simulink model "off_grid_RRC"  (R2015b)
settings: Solver=ode45  StartTime=0.0  StopTime=5  RelTol=1e-3
libraries: powerlib x55, powerlib_meascontrol x6, powerlib_extras x6
settings Model: Creator=Pouyan  LastModifiedBy=fujitsu
settings DataIOCC: SaveFormat=Array  SignalLoggingSaveFormat=ModelDataLogs
settings OptimizationCC: ExpressionDepthLimit=2147483647
settings DebuggingCC: UnderspecifiedInitializationDetection=Classic  MergeDetectMultiDrivingBlocksExec=none  SolverPrmCheckMsg=warning  FcnCallInpInsideContextMsg=UseLocalSettings  StateNameClashWarn=warning
settings HardwareCC: ProdBitPerPointer=32  ProdLargestAtomicFloat=None  ProdIntDivRoundTo=Undefined  ProdEndianess=Unspecified  ProdWordSize=32  ProdHWDeviceType=32-bit Generic
settings GRTTargetCC: GeneratePreprocessorConditionals=Disable all  CombineOutputUpdateFcns=off  GRTInterface=on
settings ConfigComp: CovModelRefEnable=Off

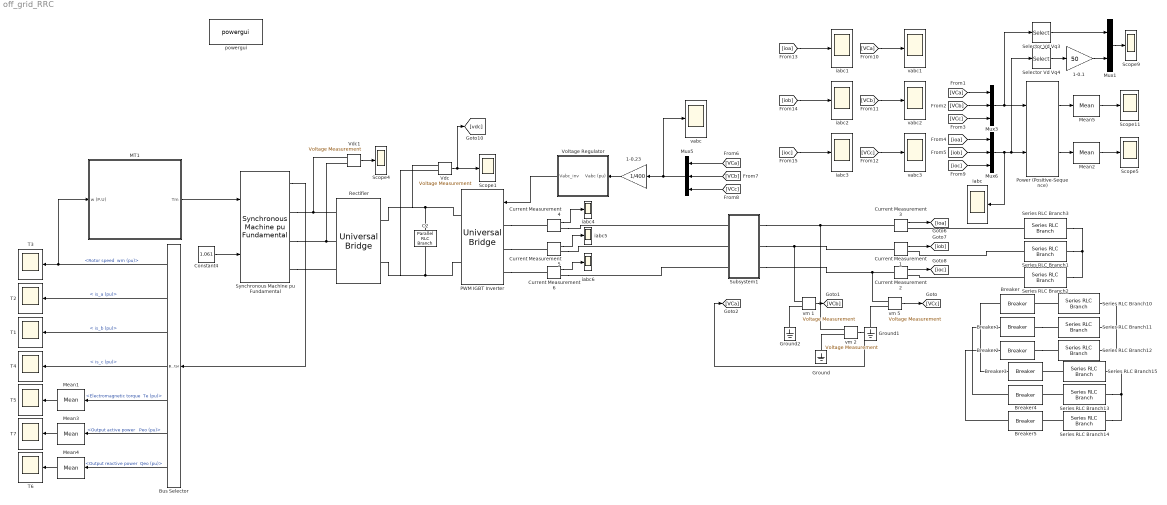
== system off_grid_RRC ==
  1-0.1 : Gain  Gain=50
  1-0.23 : Gain  Gain=1/400
  Breaker : powerlib/Elements/Breaker  InitialState=0  SwitchingTimes=[4 8]  External=off  BreakerResistance=0.01  SnubberResistance=1e6  SnubberCapacitance=inf  Measurements=None  MoreParameters=on  NoBreakLoop=off
  Breaker1 : powerlib/Elements/Breaker  InitialState=0  SwitchingTimes=[4 8]  External=off  BreakerResistance=0.01  SnubberResistance=1e6  SnubberCapacitance=inf  Measurements=None  MoreParameters=on  NoBreakLoop=off
  Breaker2 : powerlib/Elements/Breaker  InitialState=0  SwitchingTimes=[4 8]  External=off  BreakerResistance=0.01  SnubberResistance=1e6  SnubberCapacitance=inf  Measurements=None  MoreParameters=on  NoBreakLoop=off
  Breaker3 : powerlib/Elements/Breaker  InitialState=0  SwitchingTimes=[6 8.5]  External=off  BreakerResistance=0.01  SnubberResistance=1e6  SnubberCapacitance=inf  Measurements=None  MoreParameters=on  NoBreakLoop=off
  Breaker4 : powerlib/Elements/Breaker  InitialState=0  SwitchingTimes=[6 8.5]  External=off  BreakerResistance=0.01  SnubberResistance=1e6  SnubberCapacitance=inf  Measurements=None  MoreParameters=on  NoBreakLoop=off
  Breaker5 : powerlib/Elements/Breaker  InitialState=0  SwitchingTimes=[6 8.5]  External=off  BreakerResistance=0.01  SnubberResistance=1e6  SnubberCapacitance=inf  Measurements=None  MoreParameters=on  NoBreakLoop=off
  Bus Selector : BusSelector  OutputSignals="Mechanical.Rotor speed  wm (pu),Stator current. is_a (pu),Stator current. is_b (pu),Stator current. is_c (pu),Mechanical.Electromagnetic torque  Te (pu),Output active power   Peo (pu),Output reactive power  Qeo (pu)"
  C2 : powerlib/Elements/Parallel RLC Branch  LConnTagsString=a  RConnTagsString=__new0  BranchType=C  Resistance=inf  Inductance=inf  SetiL0=off  InitialCurrent=0  Capacitance=5000e-06  Setx0=off  InitialVoltage=0  Measurements=None
  Constant4 : Constant  Value=1.061
  Current Measurement{1..6} (6 alike) : powerlib/Measurements/Current Measurement  PhasorSimulation=off  OutputType=Complex  PSBequivalent=0
  Ground : powerlib/Elements/Ground  LConnTagsString=a
  Ground1 : powerlib/Elements/Ground  LConnTagsString=a
  Ground2 : powerlib/Elements/Ground  LConnTagsString=a
  MT1 : Subsystem
  Mean{1..5} (5 alike) : powerlib_meascontrol/Measurements/Mean  Freq=50  Vinit=0  Ts=5e-6
  Mux1 : Mux  Inputs=2
  Mux3 : Mux  Inputs=3
  Mux5 : Mux  Inputs=3
  Mux6 : Mux  Inputs=3
  PWM IGBT Inverter : powerlib/Power Electronics/Universal Bridge  Arms=3  SnubberResistance=5000  SnubberCapacitance=inf  Device=IGBT / Diodes  Ron=1e-3  Lon=0  ForwardVoltages="[  0.0  0.0  ]"  ForwardVoltage=.8  GTOparameters=[ 1e-6 ,1e-6 ]  IGBTparameters=[ 1e-6 , 2e-6 ]  Measurements=Device currents  Measurements_2=None  converterType=Rectifier
  Power (Positive-Sequence) : powerlib_meascontrol/Measurements/Power (Positive-Sequence)  Freq=50  Vinit=[0, 0]  Iinit=[0, 0]  Ts=5e-6
  Rectifier : powerlib/Power Electronics/Universal Bridge  Arms=3  SnubberResistance=50  SnubberCapacitance=0.1e-6  Device=Diodes  Ron=1e-3  Lon=0  ForwardVoltages="[  0.8  0.8  ]"  ForwardVoltage=.7  GTOparameters=[ 10e-6 , 20e-6 ]  IGBTparameters=[ 1e-6 , 2e-6 ]  Measurements=Device currents  Measurements_2=None  converterType=Rectifier
  Scope{1,4..5,9,11} (5 alike) : Scope
  Selector Vd Vq3 : Selector  InputPortWidth=3  IndexOptions=Index vector (dialog)  Indices=[1]  OutputSizes=1
  Selector Vd Vq4 : Selector  InputPortWidth=3  IndexOptions=Index vector (dialog)  Indices=[1]  OutputSizes=1
  Series RLC Branch1 : powerlib/Elements/Series RLC Branch  LConnTagsString=__new0  RConnTagsString=__new0  BranchType=RL  Resistance=50  Inductance=100e-3  SetiL0=off  InitialCurrent=0  Capacitance=1e-6  Setx0=off  InitialVoltage=0  Measurements=None
  Series RLC Branch10 : powerlib/Elements/Series RLC Branch  LConnTagsString=__new0  RConnTagsString=__new0  BranchType=RL  Resistance=50*2  Inductance=100e-3*2  SetiL0=off  InitialCurrent=0  Capacitance=1e-6  Setx0=off  InitialVoltage=0  Measurements=None
  Series RLC Branch11 : powerlib/Elements/Series RLC Branch  LConnTagsString=__new0  RConnTagsString=__new0  BranchType=RL  Resistance=50*2  Inductance=100e-3*2  SetiL0=off  InitialCurrent=0  Capacitance=1e-6  Setx0=off  InitialVoltage=0  Measurements=None
  Series RLC Branch12 : powerlib/Elements/Series RLC Branch  LConnTagsString=__new0  RConnTagsString=__new0  BranchType=RL  Resistance=50*2  Inductance=100e-3*2  SetiL0=off  InitialCurrent=0  Capacitance=1e-6  Setx0=off  InitialVoltage=0  Measurements=None
  Series RLC Branch13 : powerlib/Elements/Series RLC Branch  LConnTagsString=__new0  RConnTagsString=__new0  BranchType=RL  Resistance=50*3  Inductance=(100e-3)*3  SetiL0=off  InitialCurrent=0  Capacitance=1e-6  Setx0=off  InitialVoltage=0  Measurements=None
  Series RLC Branch14 : powerlib/Elements/Series RLC Branch  LConnTagsString=__new0  RConnTagsString=__new0  BranchType=RL  Resistance=50*3  Inductance=(100e-3)*3  SetiL0=off  InitialCurrent=0  Capacitance=1e-6  Setx0=off  InitialVoltage=0  Measurements=None
  Series RLC Branch15 : powerlib/Elements/Series RLC Branch  LConnTagsString=__new0  RConnTagsString=__new0  BranchType=RL  Resistance=50*3  Inductance=(100e-3)*3  SetiL0=off  InitialCurrent=0  Capacitance=1e-6  Setx0=off  InitialVoltage=0  Measurements=None
  Series RLC Branch2 : powerlib/Elements/Series RLC Branch  LConnTagsString=__new0  RConnTagsString=__new0  BranchType=RL  Resistance=50  Inductance=100e-3  SetiL0=off  InitialCurrent=0  Capacitance=1e-6  Setx0=off  InitialVoltage=0  Measurements=None
  Series RLC Branch3 : powerlib/Elements/Series RLC Branch  LConnTagsString=__new0  RConnTagsString=__new0  BranchType=RL  Resistance=50  Inductance=100e-3  SetiL0=off  InitialCurrent=0  Capacitance=1e-6  Setx0=off  InitialVoltage=0  Measurements=None
  Subsystem1 : Subsystem
  Synchronous Machine pu Fundamental : powerlib/Machines/Synchronous Machine pu Fundamental  PresetModel=No  MechanicalLoad=Mechanical power Pm  ShowDetailedParameters=on  RotorType=Salient-pole  Units=per unit fundamental parameters  MeasurementBus=off  NominalParameters="[ 30e3  550 1600]"  Stator="[ 0.2503  0.114  0.6875  0.6875 ]"  Field="[ 1  10e15/(100*pi)]"  Dampers2=[0.0652, 0.5134, 0.0287, 0.2553, 7.765e-3, 0.9167 ]  Dampers1="[ 1.17E-02  0.182  1.97E-02  0.384 ]"  Mechanical=[ 6 0 2]  PolePairs=20  InitialConditions="[ 0  0  0  0  0  0  0  0  1 ]"  SetSaturation=off  Saturation=[0.6404,0.7127,0.8441,0.9214,0.9956,1.082,1.19,1.316,1.457;0.7,0.7698,0.8872,0.9466,0.9969,1.046,1.1,1.151,1.201]  LoadFlowParameters=[1,0,0,0,0]  TsPowergui=0  TsBlock=-1  IterativeModel=Trapezoidal non iterative  BusType=swing  Pref=0  Qref=0  Qmin=-inf  Qmax=inf  PLF=0  QLF=0
  T{1..7} (7 alike) : Scope
  Vdc : powerlib/Measurements/Voltage Measurement  Tag=PoWeRsYsTeMmEaSuReMeNt  PhasorSimulation=off  OutputType=Magnitude  PSBequivalent=0
  Vdc1 : powerlib/Measurements/Voltage Measurement  Tag=PoWeRsYsTeMmEaSuReMeNt  PhasorSimulation=off  OutputType=Magnitude  PSBequivalent=0
  Voltage Regulator : Subsystem  mask{kp=0.0001, ki=5}
  iabc{,1..6} (7 alike) : Scope
  powergui : powerlib/powergui  SimulationMode=Discrete  SolverType=Tustin  SampleTime=5e-6  frequency=60  SPID=off  DisableSnubberDevices=off  DisableRonSwitches=off  DisableVfSwitches=off  SwTol=0  DisplayEquations=off  Interpol=off  ExternalGateDelay=off  methode=off  Ts=0  FunctionMessages=off  echomessages=off  HookPort=off  EnableUseOfTLC=off  x0status=blocks  frequencyindice=0  Pbase=100e6  ErrMax=0.0001  Iterations=50  UnitsV=kV  UnitsW=MW  buscounter=0  RestoreLinks=warning  ResistiveCurrentMeasurement=off  Frange=[0:2:500]  Ylog=off  Xlog=on  ShowGrid=off  save=off  variable=ZData  structure=Vs  ZoomFFT=on  StartTime=1/60  cycles=1  DisplayStyle=1  fundamental=60  FreqAxis=on  MaxFrequency=10000  frequencyindicesteady=1  RmsSteady=1  display=off
  vabc{,1..3} (4 alike) : Scope
  vm 1 : powerlib/Measurements/Voltage Measurement  PhasorSimulation=off  OutputType=Complex  PSBequivalent=0
  vm 2 : powerlib/Measurements/Voltage Measurement  PhasorSimulation=off  OutputType=Complex  PSBequivalent=0
  vm 5 : powerlib/Measurements/Voltage Measurement  PhasorSimulation=off  OutputType=Complex  PSBequivalent=0
  wires:
  Power (Positive-Sequence)/1 -> Mean5/1
  Mean5/1 -> Scope11/1
  Mean2/1 -> Scope5/1
  MT1/1(Tm) -> Synchronous Machine pu Fundamental/1
  Synchronous Machine pu Fundamental/1 -> Bus Selector/1
  Constant4/1 -> Synchronous Machine pu Fundamental/2
  Vdc1/1 -> Scope4/1
  Vdc/1 -> [vdc], Scope1/1
  Voltage Regulator/1(Vabc_inv) -> PWM IGBT Inverter/1
  Mux1/1 -> Scope9/1
  Selector Vd Vq3/1 -> Mux1/1
  Mean4/1 -> T6/1
  Bus Selector/1 -> MT1/1(w (P.U)), T3/1  "<Rotor speed  wm (pu)>"
  Bus Selector/2 -> T2/1  "< is_a (pu)>"
  Bus Selector/3 -> T1/1  "< is_b (pu)>"
  Bus Selector/4 -> T4/1  "< is_c (pu)>"
  Bus Selector/5 -> Mean1/1  "<Electromagnetic torque  Te (pu)>"
  Mean1/1 -> T5/1
  Bus Selector/7 -> Mean4/1  "<Output reactive power  Qeo (pu)>"
  Bus Selector/6 -> Mean3/1  "<Output active power   Peo (pu)>"
  Mean3/1 -> T7/1
  Power (Positive-Sequence)/2 -> Mean2/1
  vm 5/1 -> [VCc]
  vm 1/1 -> [VCb]
  vm 2/1 -> [VCa]
  Current Measurement2/1 -> [ioc]
  1-0.23/1 -> Voltage Regulator/1(Vabc (pu))
  [VCa] -> Mux5/1
  [VCb] -> Mux5/2
  [VCc] -> Mux5/3
  Mux5/1 -> vabc/1, 1-0.23/1
  [VCc] -> Mux3/3
  [VCa] -> Mux3/1
  [VCb] -> Mux3/2
  Mux3/1 -> Selector Vd Vq3/1, Power (Positive-Sequence)/1
  [ioa] -> Mux6/1
  [iob] -> Mux6/2
  [ioc] -> Mux6/3
  Mux6/1 -> iabc/1, Selector Vd Vq4/1, Power (Positive-Sequence)/2
  Current Measurement1/1 -> [iob]
  Current Measurement3/1 -> [ioa]
  [VCa] -> vabc1/1
  [VCb] -> vabc2/1
  [VCc] -> vabc3/1
  [ioa] -> iabc1/1
  [iob] -> iabc2/1
  [ioc] -> iabc3/1
  Current Measurement4/1 -> iabc4/1
  Current Measurement5/1 -> iabc5/1
  Current Measurement6/1 -> iabc6/1
  Selector Vd Vq4/1 -> 1-0.1/1
  1-0.1/1 -> Mux1/2
  connections:
  Synchronous Machine pu Fundamental/RConn1 -- Vdc1/LConn1 -- Rectifier/LConn1
  Synchronous Machine pu Fundamental/RConn2 -- Rectifier/LConn2 -- Vdc1/LConn2
  Synchronous Machine pu Fundamental/RConn3 -- Rectifier/LConn3
  Series RLC Branch3/RConn1 -- Series RLC Branch2/RConn1 -- Series RLC Branch1/RConn1
  Series RLC Branch10/RConn1 -- Series RLC Branch12/RConn1 -- Series RLC Branch11/RConn1
  Series RLC Branch3/LConn1 -- Current Measurement3/RConn1
  Series RLC Branch1/LConn1 -- Current Measurement1/RConn1
  Series RLC Branch2/LConn1 -- Current Measurement2/RConn1
  Series RLC Branch10/LConn1 -- Breaker/RConn1
  Breaker1/RConn1 -- Series RLC Branch11/LConn1
  Breaker2/RConn1 -- Series RLC Branch12/LConn1
  Current Measurement4/RConn1 -- Subsystem1/LConn1
  PWM IGBT Inverter/LConn1 -- Current Measurement4/LConn1
  Current Measurement5/RConn1 -- Subsystem1/LConn2
  PWM IGBT Inverter/LConn2 -- Current Measurement5/LConn1
  Current Measurement6/RConn1 -- Subsystem1/LConn3
  PWM IGBT Inverter/LConn3 -- Current Measurement6/LConn1
  Series RLC Branch15/RConn1 -- Series RLC Branch14/RConn1 -- Series RLC Branch13/RConn1
  Series RLC Branch15/LConn1 -- Breaker3/RConn1
  Series RLC Branch13/LConn1 -- Breaker4/RConn1
  Series RLC Branch14/LConn1 -- Breaker5/RConn1
  Rectifier/RConn2 -- Vdc/LConn2 -- PWM IGBT Inverter/RConn2 -- C2/RConn1
  PWM IGBT Inverter/RConn1 -- Rectifier/RConn1 -- Vdc/LConn1 -- C2/LConn1
  Breaker5/LConn1 -- Breaker2/LConn1
  Breaker4/LConn1 -- Breaker1/LConn1
  Breaker/LConn1 -- Breaker3/LConn1
  Subsystem1/RConn1 -- Current Measurement3/LConn1 -- vm 2/LConn1
  Subsystem1/RConn2 -- vm 1/LConn1 -- Current Measurement1/LConn1
  Subsystem1/RConn3 -- vm 5/LConn1 -- Current Measurement2/LConn1
  vm 2/LConn2 -- Ground/LConn1
  vm 5/LConn2 -- Ground1/LConn1
  vm 1/LConn2 -- Ground2/LConn1

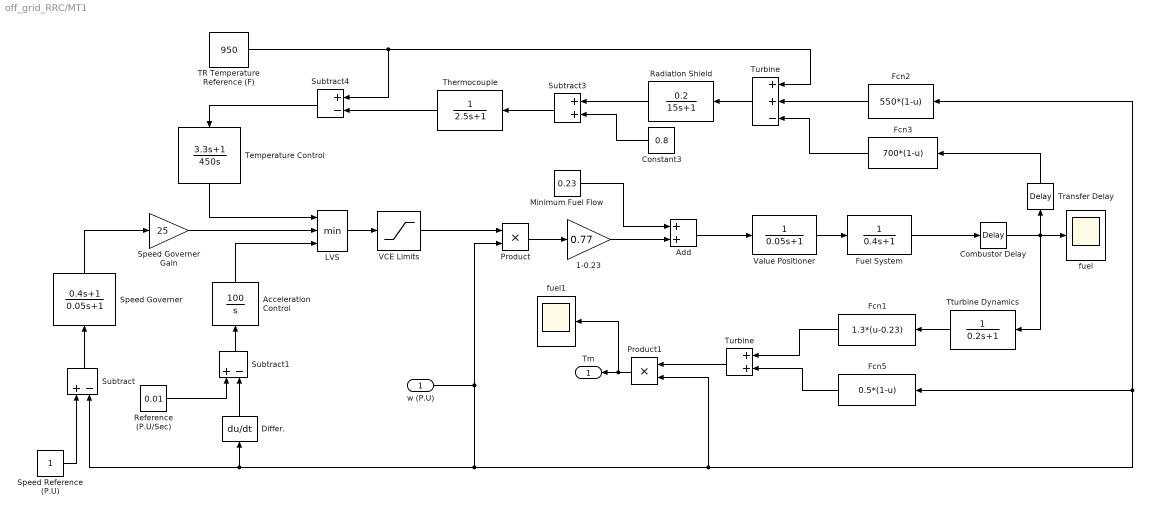
== system off_grid_RRC/MT1 ==
  w (P.U) : Inport
  1-0.23 : Gain  Gain=0.77
  Acceleration Control : TransferFcn  Numerator=[0 100]  Denominator=[1 0]
  Add : Sum
  Combustor Delay : TransportDelay  DelayTime=0.01
  Constant3 : Constant  Value=0.8
  Differ. : Derivative
  Fcn1 : Fcn  Expr=1.3*(u-0.23)
  Fcn2 : Fcn  Expr=550*(1-u)
  Fcn3 : Fcn  Expr=700*(1-u)
  Fcn5 : Fcn  Expr=0.5*(1-u)
  Fuel System : TransferFcn  Denominator=[0.4 1]
  LVS : MinMax  Inputs=3
  Minimum Fuel Flow : Constant  Value=0.23
  Product : Product  RndMeth=Zero
  Product1 : Product  RndMeth=Zero
  Radiation Shield : TransferFcn  Numerator=[0.2]  Denominator=[15 1]
  Reference (P.U/Sec) : Constant  Value=0.01
  Speed Governer : TransferFcn  Numerator=[0.4 1]  Denominator=[0.05 1]
  Speed Governer Gain : Gain  Gain=25
  Speed Reference (P.U) : Constant
  Subtract : Sum  Inputs=+-
  Subtract1 : Sum  Inputs=+-
  Subtract3 : Sum
  Subtract4 : Sum  Inputs=+-
  TR Temperature Reference (F) : Constant  Value=950
  Temperature Control : TransferFcn  Numerator=[3.3 1]  Denominator=[450 0]
  Thermocouple : TransferFcn  Denominator=[2.5 1]
  Transfer Delay : TransportDelay  DelayTime=0.04
  Tturbine Dynamics : TransferFcn  Denominator=[0.2 1]
  Turbine : Sum  Inputs=++-
  "Turbine " : Sum
  VCE Limits : Saturate  UpperLimit=1.5  LowerLimit=-0.1
  Value Positioner : TransferFcn  Denominator=[0.05 1]
  fuel : Scope
  fuel1 : Scope
  Tm : Outport
  wires:
  "Turbine "/1 -> Product1/1
  Product1/1 -> fuel1/1, Tm/1
  Fcn5/1 -> "Turbine "/2
  Fcn1/1 -> "Turbine "/1
  Tturbine Dynamics/1 -> Fcn1/1
  w (P.U)/1 -> Fcn2/1, Fcn5/1, Product1/2, Differ./1, Subtract/2, Product/2
  Speed Governer/1 -> Speed Governer Gain/1
  Temperature Control/1 -> LVS/1
  Subtract4/1 -> Temperature Control/1
  TR Temperature Reference (F)/1 -> Subtract4/1, Turbine/1
  Thermocouple/1 -> Subtract4/2
  Subtract3/1 -> Thermocouple/1
  Turbine/1 -> Radiation Shield/1
  Constant3/1 -> Subtract3/2
  Radiation Shield/1 -> Subtract3/1
  Fcn2/1 -> Turbine/2
  Fcn3/1 -> Turbine/3
  Transfer Delay/1 -> Fcn3/1
  LVS/1 -> VCE Limits/1
  Acceleration Control/1 -> LVS/3
  Subtract1/1 -> Acceleration Control/1
  Reference (P.U/Sec)/1 -> Subtract1/1
  Differ./1 -> Subtract1/2
  Speed Governer Gain/1 -> LVS/2
  Combustor Delay/1 -> Tturbine Dynamics/1, fuel/1, Transfer Delay/1
  Fuel System/1 -> Combustor Delay/1
  Value Positioner/1 -> Fuel System/1
  Add/1 -> Value Positioner/1
  Minimum Fuel Flow/1 -> Add/1
  1-0.23/1 -> Add/2
  Product/1 -> 1-0.23/1
  VCE Limits/1 -> Product/1
  Subtract/1 -> Speed Governer/1
  Speed Reference (P.U)/1 -> Subtract/1

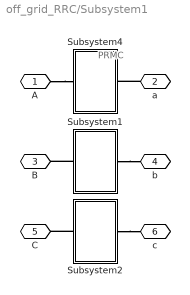
== system off_grid_RRC/Subsystem1 ==
  note: PRMC
  Subsystem1 : Subsystem
  Subsystem2 : Subsystem
  Subsystem4 : Subsystem
  A : PMIOPort  Port=1  Side=Left
  a : PMIOPort  Port=2  Side=Right
  B : PMIOPort  Port=3  Side=Left
  b : PMIOPort  Port=4  Side=Right
  C : PMIOPort  Port=5  Side=Left
  c : PMIOPort  Port=6  Side=Right
  connections:
  A/RConn1 -- Subsystem4/LConn1
  a/RConn1 -- Subsystem4/RConn1
  Subsystem1/LConn1 -- B/RConn1
  Subsystem1/RConn1 -- b/RConn1
  Subsystem2/LConn1 -- C/RConn1
  Subsystem2/RConn1 -- c/RConn1

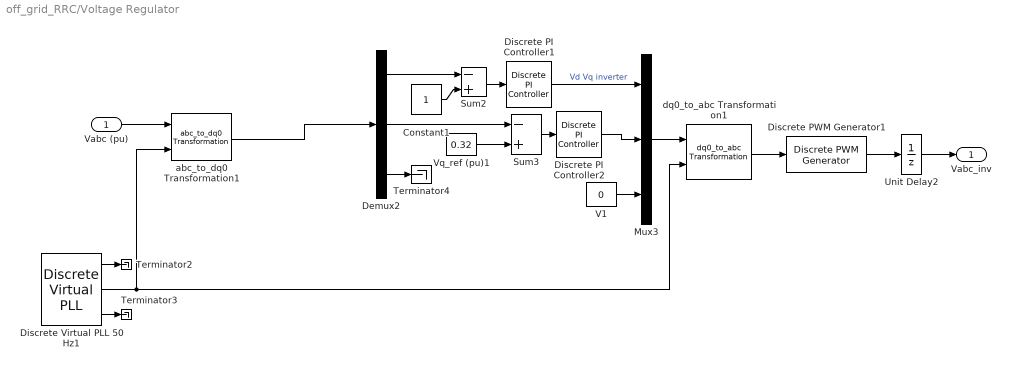
== system off_grid_RRC/Voltage Regulator ==
  Vabc (pu) : Inport
  Constant1 : Constant
  Demux2 : Demux  Outputs=3
  Discrete PI Controller1 : powerlib_extras/Discrete  Control Blocks/Discrete PI Controller  Kp=kp  Ki=ki  Par_Limits=[1 -1]  Init=0  Ts=5e-6
  Discrete PI Controller2 : powerlib_extras/Discrete  Control Blocks/Discrete PI Controller  Kp=kp  Ki=ki  Par_Limits=[1 -1]  Init=0  Ts=5e-6
  Discrete PWM Generator1 : powerlib_extras/Discrete  Control Blocks/Discrete PWM Generator  GeneratorMode="3-arm  bridge (6 pulses)"  Fc=2000  Ts=5e-6  Internal=off  mIndex=0.4  Freq=60  Phase=0
  Discrete Virtual PLL 50 Hz1 : powerlib_extras/Discrete  Control Blocks/Discrete Virtual PLL  Freq=50  Phase=0  Ts=5e-6
  Mux3 : Mux  Inputs=3
  Sum2 : Sum  Inputs=-+  SaturateOnIntegerOverflow=on  InputSameDT=on  OutDataTypeStr=Inherit: Same as first input
  Sum3 : Sum  Inputs=-+  SaturateOnIntegerOverflow=on  InputSameDT=on  OutDataTypeStr=Inherit: Same as first input
  Terminator2 : Terminator
  Terminator3 : Terminator
  Terminator4 : Terminator
  Unit Delay2 : UnitDelay  SampleTime=5e-6
  V1 : Constant  Value=0
  Vq_ref (pu)1 : Constant  Value=0.32
  abc_to_dq0 Transformation1 : powerlib_extras/Measurements/abc_to_dq0 Transformation
  dq0_to_abc Transformation1 : powerlib_extras/Measurements/dq0_to_abc Transformation
  Vabc_inv : Outport
  wires:
  Demux2/1 -> Sum2/1
  Sum2/1 -> Discrete PI Controller1/1
  Mux3/1 -> dq0_to_abc Transformation1/1
  Discrete Virtual PLL 50 Hz1/2 -> abc_to_dq0 Transformation1/2, dq0_to_abc Transformation1/2
  Discrete Virtual PLL 50 Hz1/1 -> Terminator2/1
  Discrete Virtual PLL 50 Hz1/3 -> Terminator3/1
  Discrete PWM Generator1/1 -> Unit Delay2/1
  abc_to_dq0 Transformation1/1 -> Demux2/1
  Demux2/3 -> Terminator4/1
  Constant1/1 -> Sum2/2
  Demux2/2 -> Sum3/1
  Vq_ref (pu)1/1 -> Sum3/2
  Sum3/1 -> Discrete PI Controller2/1
  Discrete PI Controller1/1 -> Mux3/1  "Vd Vq inverter"
  Discrete PI Controller2/1 -> Mux3/2
  V1/1 -> Mux3/3
  Unit Delay2/1 -> Vabc_inv/1
  Vabc (pu)/1 -> abc_to_dq0 Transformation1/1
  dq0_to_abc Transformation1/1 -> Discrete PWM Generator1/1

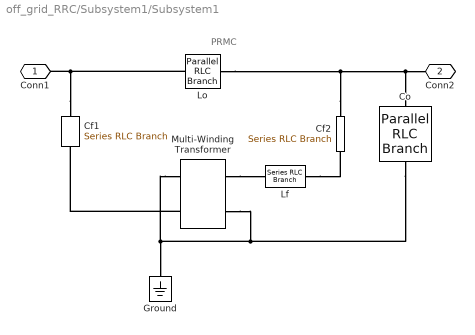
== system off_grid_RRC/Subsystem1/Subsystem1 ==
  note: PRMC
  Cf1 : powerlib/Elements/Series RLC Branch  LConnTagsString=__new0  RConnTagsString=__new0  BranchType=C  Resistance=1  Inductance=1e-3  SetiL0=off  InitialCurrent=0  Capacitance=150e-6  Setx0=off  InitialVoltage=0  Measurements=None
  Cf2 : powerlib/Elements/Series RLC Branch  LConnTagsString=__new0  RConnTagsString=__new0  BranchType=C  Resistance=1  Inductance=1e-3  SetiL0=off  InitialCurrent=0  Capacitance=150e-6  Setx0=off  InitialVoltage=0  Measurements=None
  Co : powerlib/Elements/Parallel RLC Branch  LConnTagsString=a  RConnTagsString=__new0  BranchType=C  Resistance=1  Inductance=1e-3  SetiL0=off  InitialCurrent=0  Capacitance=1.9e-5  Setx0=off  InitialVoltage=0  Measurements=None
  Ground : powerlib/Elements/Ground  LConnTagsString=a
  Lf : powerlib/Elements/Series RLC Branch  LConnTagsString=__new0  RConnTagsString=__new0  BranchType=L  Resistance=1  Inductance=800e-6  SetiL0=off  InitialCurrent=0  Capacitance=1e-6  Setx0=off  InitialVoltage=0  Measurements=None
  Lo : powerlib/Elements/Parallel RLC Branch  LConnTagsString=a  RConnTagsString=__new0  BranchType=L  Resistance=1  Inductance=0.03333  SetiL0=off  InitialCurrent=0  Capacitance=1e-6  Setx0=off  InitialVoltage=0  Measurements=None
  Multi-Winding Transformer : powerlib/Elements/Multi-Winding Transformer  LeftWindings=1  RightWindings=1  TappedWindings=no taps  NumberOfTaps=2  UNITS=pu  NominalPower=[10 60]  NominalVoltages="[100 20  120 120 ]"  WindingResistances="[ 0.0005  0.005  0.005  0.005]"  WindingInductances="[ 0.002  0.02  0.02  0.02 ]"  SetSaturation=off  Rm=25  Lm=50  Saturation=[ 0,0 ; 0.0024,1.2 ; 1.0,1.52 ]  Hysteresis=off  DataFile='hysteresis.mat'  Measurements=None  MoreParameters=off  BreakLoop=off  DataType=off  InitialFlux=0  TransfoNumber=1
  Conn1 : PMIOPort  Port=1  Side=Left
  Conn2 : PMIOPort  Port=2  Side=Right
  connections:
  Multi-Winding Transformer/LConn2 -- Cf1/RConn1
  Multi-Winding Transformer/LConn1 -- Ground/LConn1 -- Co/RConn1 -- Multi-Winding Transformer/RConn2
  Multi-Winding Transformer/RConn1 -- Lf/LConn1
  Lf/RConn1 -- Cf2/RConn1
  Cf1/LConn1 -- Conn1/RConn1 -- Lo/LConn1
  Cf2/LConn1 -- Conn2/RConn1 -- Co/LConn1 -- Lo/RConn1

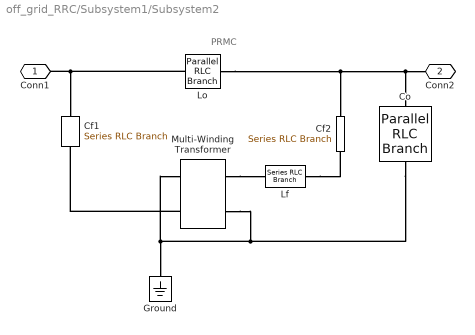
== system off_grid_RRC/Subsystem1/Subsystem2 ==
  note: PRMC
  Cf1 : powerlib/Elements/Series RLC Branch  LConnTagsString=__new0  RConnTagsString=__new0  BranchType=C  Resistance=1  Inductance=1e-3  SetiL0=off  InitialCurrent=0  Capacitance=150e-6  Setx0=off  InitialVoltage=0  Measurements=None
  Cf2 : powerlib/Elements/Series RLC Branch  LConnTagsString=__new0  RConnTagsString=__new0  BranchType=C  Resistance=1  Inductance=1e-3  SetiL0=off  InitialCurrent=0  Capacitance=150e-6  Setx0=off  InitialVoltage=0  Measurements=None
  Co : powerlib/Elements/Parallel RLC Branch  LConnTagsString=a  RConnTagsString=__new0  BranchType=C  Resistance=1  Inductance=1e-3  SetiL0=off  InitialCurrent=0  Capacitance=1.9e-5  Setx0=off  InitialVoltage=0  Measurements=None
  Ground : powerlib/Elements/Ground  LConnTagsString=a
  Lf : powerlib/Elements/Series RLC Branch  LConnTagsString=__new0  RConnTagsString=__new0  BranchType=L  Resistance=1  Inductance=800e-6  SetiL0=off  InitialCurrent=0  Capacitance=1e-6  Setx0=off  InitialVoltage=0  Measurements=None
  Lo : powerlib/Elements/Parallel RLC Branch  LConnTagsString=a  RConnTagsString=__new0  BranchType=L  Resistance=1  Inductance=0.03333  SetiL0=off  InitialCurrent=0  Capacitance=1e-6  Setx0=off  InitialVoltage=0  Measurements=None
  Multi-Winding Transformer : powerlib/Elements/Multi-Winding Transformer  LeftWindings=1  RightWindings=1  TappedWindings=no taps  NumberOfTaps=2  UNITS=pu  NominalPower=[10 60]  NominalVoltages="[100 20  120 120 ]"  WindingResistances="[ 0.0005  0.005  0.005  0.005]"  WindingInductances="[ 0.002  0.02  0.02  0.02 ]"  SetSaturation=off  Rm=25  Lm=50  Saturation=[ 0,0 ; 0.0024,1.2 ; 1.0,1.52 ]  Hysteresis=off  DataFile='hysteresis.mat'  Measurements=None  MoreParameters=off  BreakLoop=off  DataType=off  InitialFlux=0  TransfoNumber=1
  Conn1 : PMIOPort  Port=1  Side=Left
  Conn2 : PMIOPort  Port=2  Side=Right
  connections:
  Lo/RConn1 -- Co/LConn1 -- Conn2/RConn1 -- Cf2/LConn1
  Lo/LConn1 -- Conn1/RConn1 -- Cf1/LConn1
  Lf/RConn1 -- Cf2/RConn1
  Multi-Winding Transformer/RConn1 -- Lf/LConn1
  Multi-Winding Transformer/RConn2 -- Co/RConn1 -- Ground/LConn1 -- Multi-Winding Transformer/LConn1
  Multi-Winding Transformer/LConn2 -- Cf1/RConn1

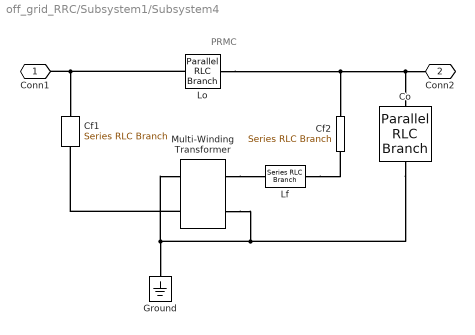
== system off_grid_RRC/Subsystem1/Subsystem4 ==
  note: PRMC
  Cf1 : powerlib/Elements/Series RLC Branch  LConnTagsString=__new0  RConnTagsString=__new0  BranchType=C  Resistance=1  Inductance=1e-3  SetiL0=off  InitialCurrent=0  Capacitance=150e-6  Setx0=off  InitialVoltage=0  Measurements=None
  Cf2 : powerlib/Elements/Series RLC Branch  LConnTagsString=__new0  RConnTagsString=__new0  BranchType=C  Resistance=1  Inductance=1e-3  SetiL0=off  InitialCurrent=0  Capacitance=150e-6  Setx0=off  InitialVoltage=0  Measurements=None
  Co : powerlib/Elements/Parallel RLC Branch  LConnTagsString=a  RConnTagsString=__new0  BranchType=C  Resistance=1  Inductance=1e-3  SetiL0=off  InitialCurrent=0  Capacitance=1.9e-5  Setx0=off  InitialVoltage=0  Measurements=None
  Ground : powerlib/Elements/Ground  LConnTagsString=a
  Lf : powerlib/Elements/Series RLC Branch  LConnTagsString=__new0  RConnTagsString=__new0  BranchType=L  Resistance=1  Inductance=800e-6  SetiL0=off  InitialCurrent=0  Capacitance=1e-6  Setx0=off  InitialVoltage=0  Measurements=None
  Lo : powerlib/Elements/Parallel RLC Branch  LConnTagsString=a  RConnTagsString=__new0  BranchType=L  Resistance=1  Inductance=0.03333  SetiL0=off  InitialCurrent=0  Capacitance=1e-6  Setx0=off  InitialVoltage=0  Measurements=None
  Multi-Winding Transformer : powerlib/Elements/Multi-Winding Transformer  LeftWindings=1  RightWindings=1  TappedWindings=no taps  NumberOfTaps=2  UNITS=pu  NominalPower=[10 60]  NominalVoltages="[100 20  120 120 ]"  WindingResistances="[ 0.0005  0.005  0.005  0.005]"  WindingInductances="[ 0.002  0.02  0.02  0.02 ]"  SetSaturation=off  Rm=25  Lm=50  Saturation=[ 0,0 ; 0.0024,1.2 ; 1.0,1.52 ]  Hysteresis=off  DataFile='hysteresis.mat'  Measurements=None  MoreParameters=off  BreakLoop=off  DataType=off  InitialFlux=0  TransfoNumber=1
  Conn1 : PMIOPort  Port=1  Side=Left
  Conn2 : PMIOPort  Port=2  Side=Right
  connections:
  Lo/RConn1 -- Co/LConn1 -- Conn2/RConn1 -- Cf2/LConn1
  Lo/LConn1 -- Conn1/RConn1 -- Cf1/LConn1
  Lf/RConn1 -- Cf2/RConn1
  Multi-Winding Transformer/RConn1 -- Lf/LConn1
  Multi-Winding Transformer/RConn2 -- Co/RConn1 -- Ground/LConn1 -- Multi-Winding Transformer/LConn1
  Multi-Winding Transformer/LConn2 -- Cf1/RConn1
